simulink model "demoMarinerPathFollowingCourseControl"  (R2024a)
settings: Solver=ode4  StartTime=0.0  StopTime=5000  FixedStep=0.1  RelTol=1e-3  EnableMultiTasking=on
model workspace (MAT data in the model file):
  h_samp = 0.5
libraries: mssSimulink x7, simulink_extras x3
settings Model: Creator=Thor  LastModifiedBy=liamz
settings SolverCC: AlgebraicLoopSolver=TrustRegion  AutoInsertRateTranBlk=on
settings DataIOCC: LimitDataPoints=on  SaveFormat=Array  SignalLoggingSaveFormat=ModelDataLogs  SignalLoggingName=sigsOut
settings OptimizationCC: BooleanDataType=off  ExpressionDepthLimit=2147483647  InitFltsAndDblsToZero=on  LifeSpan=inf
settings DebuggingCC: SaveWithParameterizedLinksMsg=none  UnderspecifiedInitializationDetection=Classic  MergeDetectMultiDrivingBlocksExec=none  SignalResolutionControl=TryResolveAllWithWarning  MultiTaskDSMMsg=warning  MultiTaskCondExecSysMsg=none  FcnCallInpInsideContextMsg=warning  UnconnectedInputMsg=warning  UnconnectedOutputMsg=warning  UnconnectedLineMsg=warning  StateNameClashWarn=warning  SFUnexpectedBacktrackingDiag=warning  SFNoUnconditionalDefaultTransitionDiag=warning  SFExecutionAtInitializationDiag=none  ArithmeticOperatorsInVariantConditions=warning
settings HardwareCC: ProdBitPerPointer=32  ProdBitPerSizeT=32  ProdBitPerPtrDiffT=32  ProdLargestAtomicFloat=None  ProdIntDivRoundTo=Undefined  ProdEndianess=Unspecified  ProdWordSize=32  ProdHWDeviceType=32-bit Generic  TargetUnknown=on
settings ModelReferenceCC: EnableRefExpFcnMdlSchedulingChecks=on  PropagateSignalLabelsOutOfModel=off
settings SFSimCC: SimUseLocalCustomCode=off  CustomCodeUndefinedFunction=UseInterfaceOnly
settings RTWCC: RTWUseLocalCustomCode=off  GPUComputeCapability=3.5  DLArmComputeVersion=19.05
settings CodeAppCC: StateflowObjectComments=on
settings GRTTargetCC: TargetFcnLib=ansi_tfl_tmw.mat  TargetLangStandard=C89/C90 (ANSI)  ModelReferenceCompliant=off  CombineOutputUpdateFcns=off  MatFileLogging=off  GRTInterface=on
settings ConfigComp: CovMetricSettings=dw  CovSaveCumulativeToWorkspaceVar=on  CovSaveSingleToWorkspaceVar=on  CovExternalEMLEnable=off

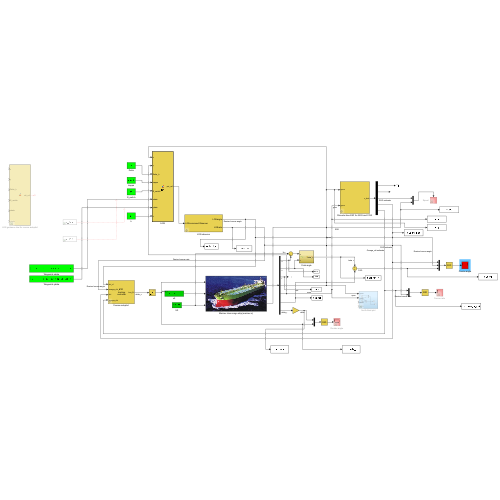
[thumbnail: Simulink's stored preview of the top-level diagram]
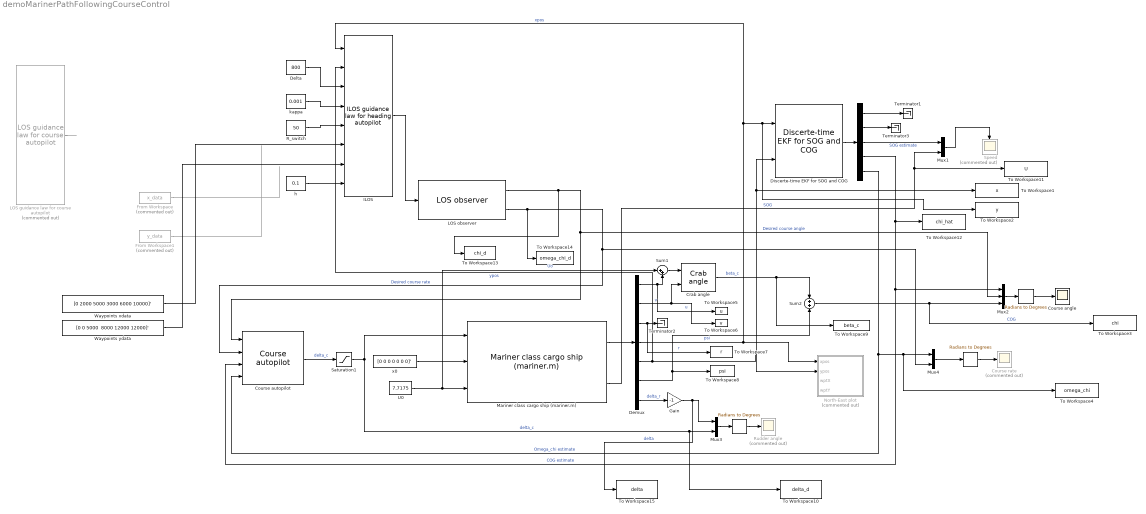
== system demoMarinerPathFollowingCourseControl ==
  "  " : simulink_extras/Transformations/Radians to Degrees
  "      " : simulink_extras/Transformations/Radians to Degrees
  "           " : simulink_extras/Transformations/Radians to Degrees
  "            " : Demux  Outputs=5
  Course angle : Scope
  "Course autopilot " : mssSimulink/Control/Autopilots/Course autopilot   T_nomoto=107.3  K_nomoto=0.185  Kp=1.45*0.9  Td=36  Ti=200
  "Course rate " : Scope  Commented=on
  Crab angle : mssSimulink/Modelling/Kinematics/Crab angle  SystemSampleTime=-1  VariantActivationTime=update diagram  AllowFlexibleInterface=on  Latency=0  AutoFrameSizeCalculation=off
  Delta : Constant  Value=800
  Demux : Demux  Outputs=7
  Discerte-time EKF for SOG and COG : mssSimulink/Navigation/Estimators/Discerte-time EKF for SOG and COG  alpha_1=0.00001  alpha_2=0.00001  Qd=100*diag([0.1,0.1])  Rd=0.1*diag([1 1])  h_samp=0.1
  From Workspace : FromWorkspace  Commented=on  VariableName=x_data
  From Workspace1 : FromWorkspace  Commented=on  VariableName=y_data
  Gain : Gain  Gain=-1
  ILOS : mssSimulink/Guidance/ILOS guidance law for heading autopilot  SystemSampleTime=-1  VariantActivationTime=update diagram  AllowFlexibleInterface=on  Latency=0  AutoFrameSizeCalculation=off
  LOS guidance law for course autopilot : mssSimulink/Guidance/LOS guidance law for course autopilot  Commented=on  SystemSampleTime=-1  VariantActivationTime=update diagram  AllowFlexibleInterface=on  Latency=0  AutoFrameSizeCalculation=off
  LOS observer : mssSimulink/Guidance/LOS observer  K_f=0.4  alpha=5
  Mariner class cargo ship (mariner.m) : mssSimulink/Marine craft models/Mariner class cargo ship (mariner.m)  SystemSampleTime=-1  VariantActivationTime=update diagram  AllowFlexibleInterface=on  Latency=0  AutoFrameSizeCalculation=off
  Mux1 : Mux  Inputs=2
  Mux2 : Mux  Inputs=3
  Mux3 : Mux  Inputs=2
  Mux4 : Mux  Inputs=2
  North-East plot : Subsystem  Commented=on  AncestorBlock=mssSimulink/Utilities/Visualization/North-East plot  StopFcn=|
      | x = xyplot.Data(:,1);
      | y = xyplot.Data(:,2);
      | wptX = waypoints(:,1);
      | wptY = waypoints(:,2);
      | figure(gcf);
      | plot(y,x,'b','linewidth',2);
      | hold on;
      | plot(wptY,wptX,'o','MarkerSize',15,'MarkerEdgeColor','k','MarkerFaceColor','c');
      | hold off;
      | xlabel('East (m)', 'FontSize', 14);
      | ylabel('North (m)', 'FontSize', 14);
      | title('North-East Positions (m)', 'FontSize', 14);
      | axis('equal');
      | grid;
  R_switch : Constant  Value=50
  Rudder angle : Scope  Commented=on
  Saturation1 : Saturate  UpperLimit=40*pi/180  LowerLimit=-40*pi/180
  Speed : Scope  Commented=on
  Sum1 : Sum  Inputs=|++
  Sum2 : Sum  Inputs=+|+
  Terminator1 : Terminator
  Terminator2 : Terminator
  Terminator3 : Terminator
  To Workspace1 : ToWorkspace  VariableName=x  SampleTime=-1
  To Workspace10 : ToWorkspace  VariableName=delta_d  SampleTime=-1
  To Workspace11 : ToWorkspace  VariableName=U  SampleTime=-1
  To Workspace12 : ToWorkspace  VariableName=chi_hat  SampleTime=-1
  To Workspace13 : ToWorkspace  VariableName=chi_d  SampleTime=-1
  To Workspace14 : ToWorkspace  VariableName=omega_chi_d  SampleTime=-1
  To Workspace15 : ToWorkspace  VariableName=delta  SampleTime=-1
  To Workspace2 : ToWorkspace  VariableName=y  SampleTime=-1
  To Workspace3 : ToWorkspace  VariableName=chi  SampleTime=-1
  To Workspace4 : ToWorkspace  VariableName=omega_chi  SampleTime=-1
  To Workspace5 : ToWorkspace  VariableName=u  SampleTime=-1
  To Workspace6 : ToWorkspace  VariableName=v  SampleTime=-1
  To Workspace7 : ToWorkspace  VariableName=r  SampleTime=-1
  To Workspace8 : ToWorkspace  VariableName=psi  SampleTime=-1
  To Workspace9 : ToWorkspace  VariableName=beta_c  SampleTime=-1
  U0 : Constant  Value=7.7175
  Waypoints xdata : Constant  Value=[0 2000 5000 3000 6000 10000]'
  Waypoints ydata : Constant  Value="[0 0 5000  8000 12000 12000]'"
  h : Constant  Value=0.1
  kappa : Constant  Value=0.001
  x0 : Constant  Value=[0 0 0 0 0 0 0]'
  wires:
  "  "/1 -> "Course rate "/1
  "Course autopilot "/1 -> Saturation1/1  "delta_c"
  LOS observer/1 -> To Workspace13/1, "Course autopilot "/1, Mux2/2  "Desired course angle"
  Demux/6 -> Sum2/2, To Workspace8/1  "psi"
  Mariner class cargo ship (mariner.m)/1 -> Demux/1
  U0/1 -> Sum1/1, Mariner class cargo ship (mariner.m)/3  "Uo"
  x0/1 -> Mariner class cargo ship (mariner.m)/2
  Demux/7 -> Gain/1  "delta_r"
  Demux/5 -> To Workspace1/1, Discerte-time EKF for SOG and COG/2, North-East plot/2(ypos), ILOS/2  "ypos"
  "           "/1 -> Course angle/1
  "            "/3 -> Mux1/1  "SOG estimate"
  Mux1/1 -> Speed/1
  Mux2/1 -> "           "/1
  Sum2/1 -> To Workspace3/1, Mux2/3  "COG"
  Mux4/1 -> "  "/1
  Mariner class cargo ship (mariner.m)/2 -> To Workspace11/1, Mux1/2  "SOG"
  R_switch/1 -> ILOS/5
  From Workspace/1 -> ?
  Delta/1 -> ILOS/3
  From Workspace1/1 -> ?
  "            "/1 -> Terminator1/1
  "            "/2 -> Terminator3/1
  Saturation1/1 -> To Workspace10/1, Mux3/2, Mariner class cargo ship (mariner.m)/1  "delta_c"
  LOS guidance law for course autopilot/1 -> ?
  Mux3/1 -> "      "/1
  "            "/5 -> "Course autopilot "/4, To Workspace4/1, Mux4/1  "Omega_chi estimate"
  "            "/4 -> To Workspace12/1, "Course autopilot "/3, Mux2/1  "COG estimate"
  LOS observer/2 -> To Workspace14/1, "Course autopilot "/2, Mux4/2  "Desired course rate"
  Crab angle/1 -> To Workspace9/1, Sum2/1  "beta_c"
  Demux/3 -> To Workspace7/1, Terminator2/1  "r"
  "      "/1 -> Rudder angle/1
  Discerte-time EKF for SOG and COG/1 -> "            "/1
  Demux/4 -> North-East plot/1(xpos), ILOS/1, To Workspace2/1, Discerte-time EKF for SOG and COG/1  "xpos"
  Gain/1 -> To Workspace15/1, Mux3/1  "delta"
  Demux/2 -> To Workspace6/1, Crab angle/2  "v"
  Demux/1 -> To Workspace5/1, Sum1/2  "u"
  Sum1/1 -> Crab angle/1
  h/1 -> ILOS/8
  kappa/1 -> ILOS/4
  ILOS/1 -> LOS observer/1
  Waypoints xdata/1 -> ILOS/6
  Waypoints ydata/1 -> ILOS/7

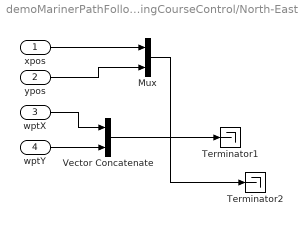
== system demoMarinerPathFollowingCourseControl/North-East plot ==
  xpos : Inport
  ypos : Inport  Port=2
  wptX : Inport  Port=3
  wptY : Inport  Port=4
  Mux : Mux  Inputs=2
  Terminator1 : Terminator
  Terminator2 : Terminator
  Vector Concatenate : Concatenate  Mode=Multidimensional array  ConcatenateDimension=2
  wires:
  wptY/1 -> Vector Concatenate/2
  wptX/1 -> Vector Concatenate/1
  xpos/1 -> Mux/1
  ypos/1 -> Mux/2
  Mux/1 -> Terminator2/1
  Vector Concatenate/1 -> Terminator1/1
